simulink model "task2b"  (R2018a)
settings: Solver=VariableStepAuto  StartTime=0.0  StopTime=40.0  RelTol=1e-3
values from neighbouring files (symbols this model uses):
  f = 1    [task2b_matlab.m]
  Gamma = [1 0 0 0 ... (first row only)    [task2b_matlab.m]
  k = 9    [task2b_matlab.m]
  lambda0 = 2    [task2b_matlab.m]
  M = 10    [task2b_matlab.m]
  p0 = 1    [task2b_matlab.m]
  sgn = sign(kp/km)    [task2b_matlab.m]
settings Model: Creator=Kristian  LastModifiedBy=Kristian

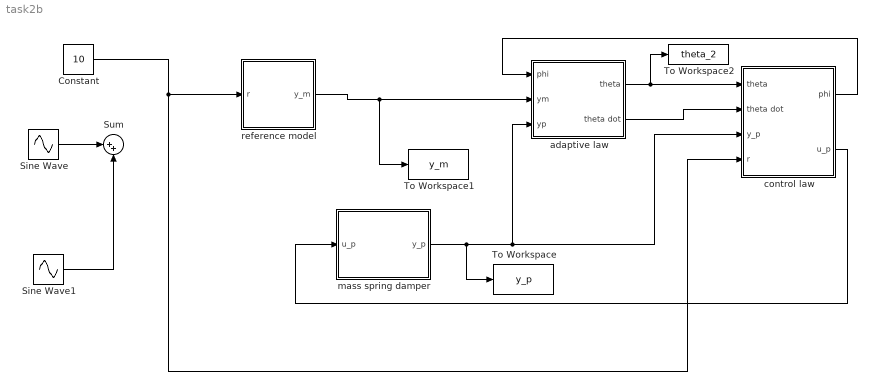
== system task2b ==
  Constant : Constant  Value=10
  Sine Wave : Sin  Amplitude=2  Frequency=3  SampleTime=0
  Sine Wave1 : Sin  Amplitude=5  SampleTime=0
  Sum : Sum  Inputs=|++
  To Workspace : ToWorkspace  VariableName=y_p  SaveFormat=Structure With Time  SampleTime=-1
  To Workspace1 : ToWorkspace  VariableName=y_m  SaveFormat=Structure With Time  SampleTime=-1
  To Workspace2 : ToWorkspace  VariableName=theta_2  SaveFormat=Structure With Time  SampleTime=-1
  adaptive law : Subsystem
  control law : Subsystem
  mass spring damper : Subsystem
  reference model : Subsystem
  wires:
  mass spring damper/1(y_p) -> To Workspace/1, adaptive law/3(yp), control law/3(y_p)
  reference model/1(y_m) -> To Workspace1/1, adaptive law/2(ym)
  adaptive law/1(theta) -> To Workspace2/1, control law/1(theta)
  adaptive law/2(theta dot) -> control law/2(theta dot)
  control law/1(phi) -> adaptive law/1(phi)
  control law/2(u_p) -> mass spring damper/1(u_p)
  Sine Wave1/1 -> Sum/2
  Sine Wave/1 -> Sum/1
  Constant/1 -> control law/4(r), reference model/1(r)

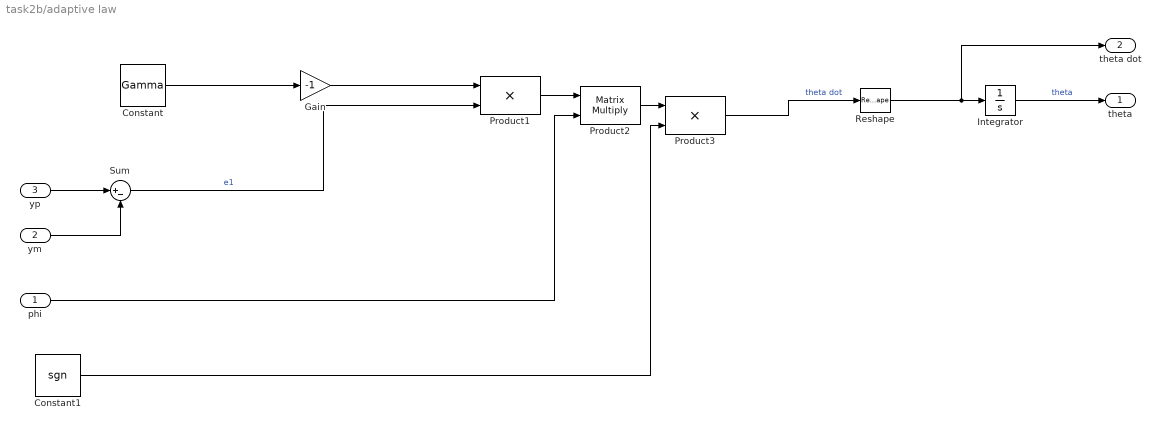
== system task2b/adaptive law ==
  phi : Inport
  ym : Inport  Port=2
  yp : Inport  Port=3
  Constant : Constant  Value=Gamma
  Constant1 : Constant  Value=sgn
  Gain : Gain  Gain=-1
  Integrator : Integrator  InitialCondition=[0; 0; 0; 0]
  Product1 : Product
  Product2 : Product  Multiplication=Matrix(*)
  Product3 : Product
  Reshape : Reshape  OutputDimensionality=Column vector (2-D)
  Sum : Sum  Inputs=|+-
  theta : Outport
  theta dot : Outport  Port=2
  wires:
  yp/1 -> Sum/1
  ym/1 -> Sum/2
  Sum/1 -> Product1/2  "e1"
  Constant/1 -> Gain/1
  Gain/1 -> Product1/1
  Product3/1 -> Reshape/1  "theta dot"
  Integrator/1 -> theta/1  "theta"
  Reshape/1 -> theta dot/1, Integrator/1
  Product1/1 -> Product2/1
  phi/1 -> Product2/2
  Product2/1 -> Product3/1
  Constant1/1 -> Product3/2

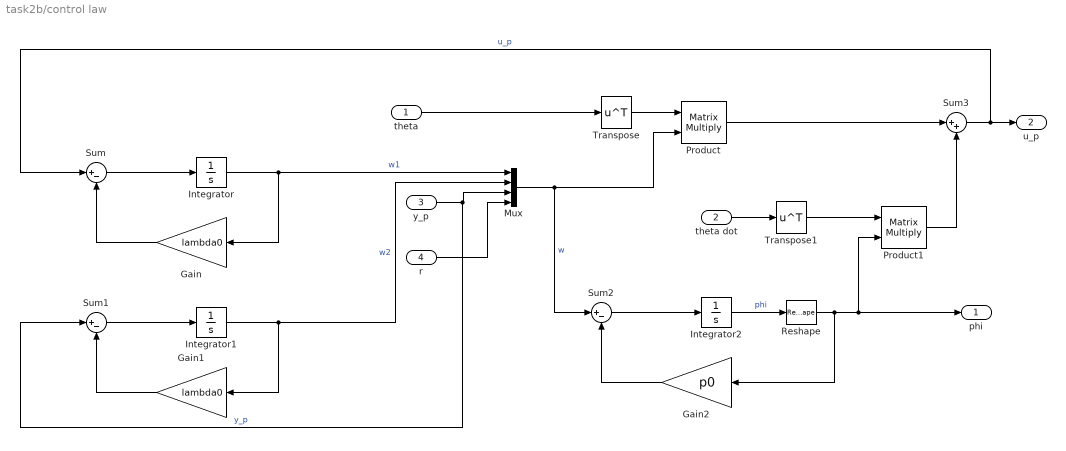
== system task2b/control law ==
  theta : Inport
  theta dot : Inport  Port=2
  y_p : Inport  Port=3
  r : Inport  Port=4
  Gain : Gain  Gain=lambda0
  Gain1 : Gain  Gain=lambda0
  Gain2 : Gain  Gain=p0
  Integrator : Integrator
  Integrator1 : Integrator
  Integrator2 : Integrator  InitialCondition=[0; 0; 0; 0]
  Mux : Mux
  Product : Product  Multiplication=Matrix(*)
  Product1 : Product  Multiplication=Matrix(*)
  Reshape : Reshape  OutputDimensionality=Column vector (2-D)
  Sum : Sum  Inputs=|+-
  Sum1 : Sum  Inputs=|+-
  Sum2 : Sum  Inputs=|+-
  Sum3 : Sum  Inputs=|++
  Transpose : Math  Operator=transpose  SaturateOnIntegerOverflow=on
  Transpose1 : Math  Operator=transpose  SaturateOnIntegerOverflow=on
  phi : Outport
  u_p : Outport  Port=2
  wires:
  Integrator/1 -> Mux/1, Gain/1  "w1"
  Sum/1 -> Integrator/1
  Gain/1 -> Sum/2
  Sum3/1 -> Sum/1, u_p/1  "u_p"
  y_p/1 -> Mux/3, Sum1/1  "y_p"
  Gain1/1 -> Sum1/2
  Integrator1/1 -> Gain1/1, Mux/2  "w2"
  Sum1/1 -> Integrator1/1
  Sum2/1 -> Integrator2/1
  Integrator2/1 -> Reshape/1  "phi"
  Gain2/1 -> Sum2/2
  Mux/1 -> Product/2, Sum2/1  "w"
  r/1 -> Mux/4
  theta/1 -> Transpose/1
  Transpose/1 -> Product/1
  Product/1 -> Sum3/1
  theta dot/1 -> Transpose1/1
  Transpose1/1 -> Product1/1
  Product1/1 -> Sum3/2
  Reshape/1 -> Product1/2, phi/1, Gain2/1

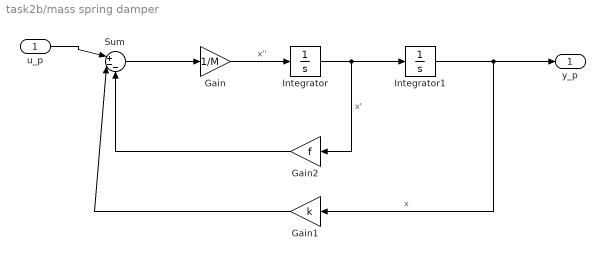
== system task2b/mass spring damper ==
  u_p : Inport
  Gain : Gain  Gain=1/M
  Gain1 : Gain  Gain=k
  Gain2 : Gain  Gain=f
  Integrator : Integrator
  Integrator1 : Integrator
  Sum : Sum  Inputs=|+--
  y_p : Outport
  wires:
  Integrator/1 -> Gain2/1, Integrator1/1  "x'"
  Sum/1 -> Gain/1
  Integrator1/1 -> y_p/1, Gain1/1  "x"
  Gain/1 -> Integrator/1  "x''"
  Gain1/1 -> Sum/2
  u_p/1 -> Sum/1
  Gain2/1 -> Sum/3

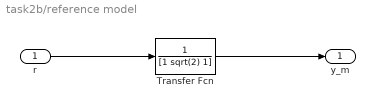
== system task2b/reference model ==
  r : Inport
  Transfer Fcn : TransferFcn  Denominator=[1 sqrt(2) 1]
  y_m : Outport
  wires:
  r/1 -> Transfer Fcn/1
  Transfer Fcn/1 -> y_m/1
